simulink model "untitled1"  (R2016a)
settings: Solver=VariableStepAuto  StartTime=0.0  StopTime=50  RelTol=1e-3
values from neighbouring files (symbols this model uses):
  K = 68.5/m    (= 0.0685)    [calculatefx0.m]
  Ka = 10    [calculatefx0.m]
  Tau = 100    [calculatefx0.m]
  TauA = 0.05    [calculatefx0.m]
  Ts = 0.25    [codeProiect.m]
  uc = 30    [calculatefx0.m]
undefined symbols (not defined in the file or in its folder): Distanta, K1, K2, K3, K4, KD_M, KI_M, KP_M
settings Model: Creator=dumea  LastModifiedBy=dumea

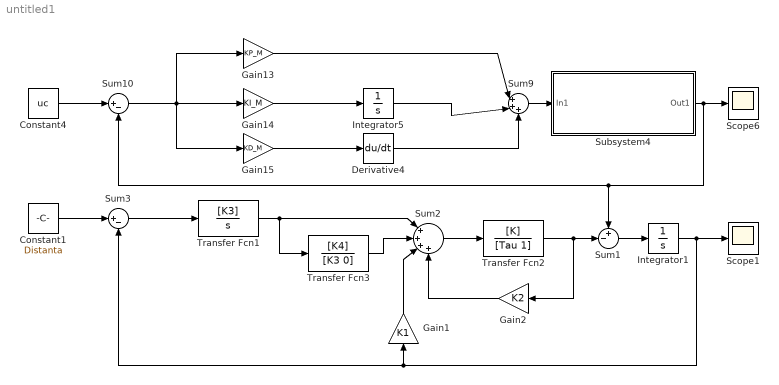
== system untitled1 ==
  Constant1 : Constant  Value=Distanta  SampleTime=Ts
  Constant4 : Constant  Value=uc
  Derivative4 : Derivative
  Gain1 : Gain  Gain=K1
  Gain13 : Gain  Gain=KP_M
  Gain14 : Gain  Gain=KI_M
  Gain15 : Gain  Gain=KD_M
  Gain2 : Gain  Gain=K2
  Integrator1 : Integrator
  Integrator5 : Integrator
  Scope1 : Scope
  Scope6 : Scope
  Subsystem4 : Subsystem
  Sum1 : Sum  Inputs=+-|
  Sum10 : Sum  Inputs=|+-
  Sum2 : Sum  Inputs=|++++
  Sum3 : Sum  Inputs=|+-
  Sum9 : Sum  Inputs=|+++
  Transfer Fcn1 : TransferFcn  Numerator=[K3]  Denominator=[1 0]
  Transfer Fcn2 : TransferFcn  Numerator=[K]  Denominator=[Tau 1]
  Transfer Fcn3 : TransferFcn  Numerator=[K4]  Denominator=[K3 0]
  wires:
  Gain15/1 -> Derivative4/1
  Derivative4/1 -> Sum9/3
  Integrator5/1 -> Sum9/2
  Gain14/1 -> Integrator5/1
  Gain13/1 -> Sum9/1
  Sum10/1 -> Gain13/1, Gain15/1, Gain14/1
  Subsystem4/1(Out1) -> Scope6/1, Sum10/2, Sum1/1
  Transfer Fcn2/1 -> Gain2/1, Sum1/2
  Sum1/1 -> Integrator1/1
  Integrator1/1 -> Scope1/1, Sum3/2, Gain1/1
  Constant1/1 -> Sum3/1
  Constant4/1 -> Sum10/1
  Sum9/1 -> Subsystem4/1(In1)
  Sum3/1 -> Transfer Fcn1/1
  Transfer Fcn1/1 -> Transfer Fcn3/1, Sum2/1
  Transfer Fcn3/1 -> Sum2/2
  Gain1/1 -> Sum2/3
  Gain2/1 -> Sum2/4
  Sum2/1 -> Transfer Fcn2/1

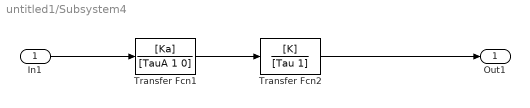
== system untitled1/Subsystem4 ==
  In1 : Inport
  Transfer Fcn1 : TransferFcn  Numerator=[Ka]  Denominator=[TauA 1 0]
  Transfer Fcn2 : TransferFcn  Numerator=[K]  Denominator=[Tau 1]
  Out1 : Outport
  wires:
  Transfer Fcn2/1 -> Out1/1
  In1/1 -> Transfer Fcn1/1
  Transfer Fcn1/1 -> Transfer Fcn2/1
